simulink model "Single_Phase_Transformer"  (R2025a)
settings: Solver=ode23tb  StartTime=0.0  StopTime=10.0  MaxStep=1e-4  RelTol=1e-3
libraries: spsRMSLib x4, spsCurrentMeasurementLib x2, spsVoltageMeasurementLib x2, spsLinearTransformerLib x1, spsACVoltageSourceLib x1, spsSeriesRLCBranchLib x1, sps_lib x1
settings Model: Creator=Jawad  LastModifiedBy=Jawad

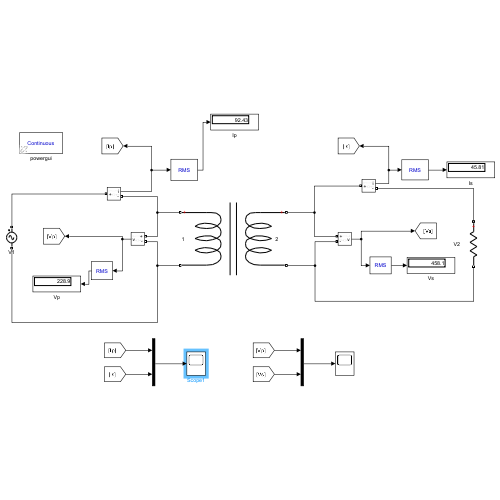
[thumbnail: Simulink's stored preview of the top-level diagram]
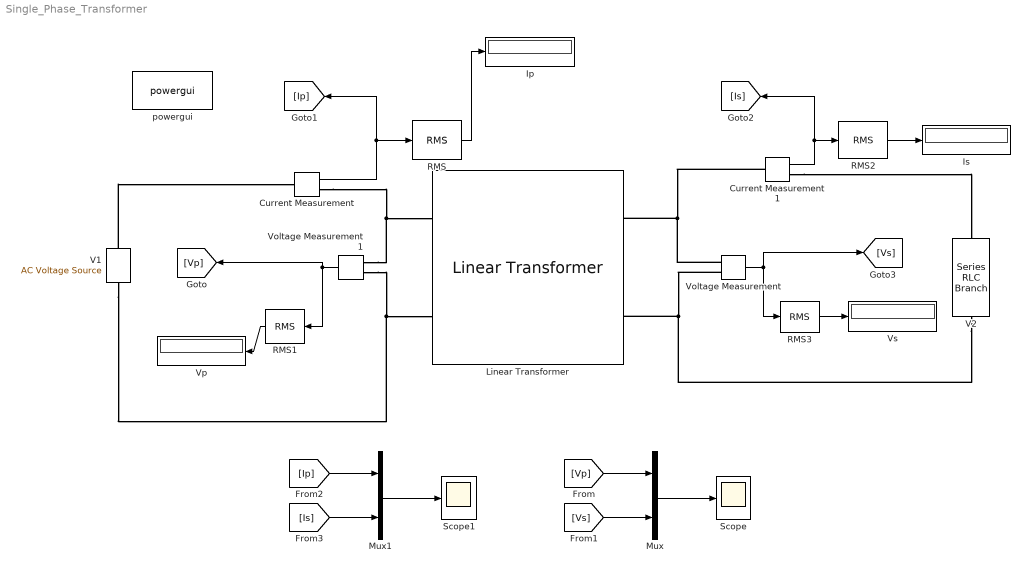
== system Single_Phase_Transformer ==
  Current Measurement : spsCurrentMeasurementLib/Current Measurement  PhasorSimulation=off  OutputType=Complex  PSBequivalent=0
  Current Measurement1 : spsCurrentMeasurementLib/Current Measurement  PhasorSimulation=off  OutputType=Complex  PSBequivalent=0
  Ip : Display
  Is : Display
  Linear Transformer : spsLinearTransformerLib/Linear Transformer  UNITS=pu  NominalPower=[ 2e6 50 ]  winding1=[400 0.002 0.08]  winding2=[800 0.002 0.08]  ThreeWindings=off  winding3=[3.15e+05 0.002 0.08]  RmLm=[4000 4000]  Measurements=None  DataType=off
  Mux : Mux  Inputs=2
  Mux1 : Mux  Inputs=2
  RMS{,1..3} (4 alike) : spsRMSLib/RMS  TrueRMS=on  Freq=60  RMSInit=120  Ts=0
  Scope : Scope
      settings: ActiveDisplayYMinimum=-882.10360137489556  ActiveDisplayYMaximum=673.27987588530846
  Scope1 : Scope
      settings: ActiveDisplayYMinimum=-156.76139668107811  ActiveDisplayYMaximum=156.76133415502477
  V1 : spsACVoltageSourceLib/AC Voltage Source  Amplitude=220*sqrt(2)  Phase=0  Frequency=50  SampleTime=0  Measurements=None  BusType=swing  Pref=10e3  Qref=0  Qmin=-inf  Qmax=+inf
  V2 : spsSeriesRLCBranchLib/Series RLC Branch  LConnTagsString=__new0  RConnTagsString=__new0  BranchType=R  Resistance=10  Inductance=1e-3  SetiL0=off  InitialCurrent=0  Capacitance=1e-6  Setx0=off  InitialVoltage=0  Measurements=None
  Voltage Measurement : spsVoltageMeasurementLib/Voltage Measurement  PhasorSimulation=off  OutputType=Complex  PSBequivalent=0
  Voltage Measurement1 : spsVoltageMeasurementLib/Voltage Measurement  PhasorSimulation=off  OutputType=Complex  PSBequivalent=0
  Vp : Display
  Vs : Display
  powergui : sps_lib/powergui  Priority=1  SimulationMode=Continuous  SampleTime=50e-6  frequency=60  Iterations=50  frequencyindice=50  Pbase=100e6  ErrMax=1e-4  UnitsV=kV  UnitsW=MW  buscounter=0  FunctionMessages=off  echomessages=off  EnableUseOfTLC=off  CurrentSourceSwitches=off  DisableSnubberDevices=off  DisableRonSwitches=off  DisableVfSwitches=off  DisplayEquations=off  AutomaticDiscreteSolvers=off  SolverType=Tustin/Backward Euler (TBE)  Interpol=off  ExternalGateDelay=off  methode=off  Ts=100  x0status=blocks  SPID=on  SwTol=0  HookPort=off  NonlinearTolerance=1e-4  nMaxIteration=100  ContinueOnMaxIteration=off  RestoreLinks=warning  ResistiveCurrentMeasurement=off  Frange=[0:2:500]  Ylog=off  Xlog=on  ShowGrid=off  save=off  variable=ZData  structure=0  ZoomFFT=off  StartTime=0.0  cycles=1  DisplayStyle=1  fundamental=60  FreqAxis=off  MaxFrequency=1000  frequencyindicesteady=1  RmsSteady=1  display=off
  wires:
  Current Measurement/1 -> [Ip], RMS/1
  RMS/1 -> Ip/1
  Voltage Measurement1/1 -> RMS1/1, [Vp]
  RMS1/1 -> Vp/1
  Current Measurement1/1 -> [Is], RMS2/1
  RMS2/1 -> Is/1
  Voltage Measurement/1 -> RMS3/1, [Vs]
  RMS3/1 -> Vs/1
  Mux/1 -> Scope/1
  [Vp] -> Mux/1
  [Vs] -> Mux/2
  [Is] -> Mux1/2
  Mux1/1 -> Scope1/1
  [Ip] -> Mux1/1
  connections:
  V1/RConn1 -- Current Measurement/LConn1
  Current Measurement/RConn1 -- Voltage Measurement1/LConn1 -- Linear Transformer/LConn1
  V1/LConn1 -- Voltage Measurement1/LConn2 -- Linear Transformer/LConn2
  Current Measurement1/LConn1 -- Voltage Measurement/LConn1 -- Linear Transformer/RConn1
  Current Measurement1/RConn1 -- V2/LConn1
  V2/RConn1 -- Voltage Measurement/LConn2 -- Linear Transformer/RConn2
